simulink model "model_22"  (R2022b)
settings: Solver=ode4  StartTime=0.0  StopTime=tfinal  FixedStep=dt  RelTol=1e-3
values from neighbouring files (symbols this model uses):
  A_mat = [A_longitudinal, zeros(size(A_longitudinal,1),size(A_lateral,2)) ... (first row only)    [pre_simulink.m]
  B_mat = [B_longitudinal, zeros(size(B_longitudinal,1),2) ... (first row only)    [pre_simulink.m]
  C_mat = eye(size(A_mat))    [pre_simulink.m]
  Controls_Matrix = [0,    XDE,   XDTH,      0 ... (first row only)    [aircraft_data_reader.m]
  D_mat = zeros(size(B_mat))    [pre_simulink.m]
  dA = 0 *pi/180    (= 0)    [pre_simulink.m]
  dE = 0 *pi/180    (= 0)    [pre_simulink.m]
  dR = 0 *pi/180    (= 0)    [pre_simulink.m]
  dTH = 0    [pre_simulink.m]
  g = aircraft_data(52)    [aircraft_data_reader.m]
  Ixx = aircraft_data(53)    [aircraft_data_reader.m]
  Iyy = aircraft_data(54)    [aircraft_data_reader.m]
  Izz = aircraft_data(55)    [aircraft_data_reader.m]
  m = aircraft_data(51)    [aircraft_data_reader.m]
  mg0 = m*g * [ sin(s0(8)) ; -cos(s0(8))*sin(s0(7)) ; -cos(s0(8))*cos(s0(7)) ]    [aircraft_data_reader.m]
  s0 = aircraft_data(4:15)    [aircraft_data_reader.m]
  States_Matrix = [XU,   0,   XW,    0,   0,   0,    0 ... (first row only)    [aircraft_data_reader.m]
  U0 = s0(1)    [aircraft_data_reader.m]
undefined symbols (not defined in the file or in its folder): A_lateral_1DOF, A_lateral_2DOF, A_lateral_3DOF_DR, A_lateral_3DOF_SP, A_longitudinal_lp, A_longitudinal_sp, alpha, B_lateral_1DOF, B_lateral_2DOF, B_lateral_3DOF_DR, B_lateral_3DOF_SP, B_longitudinal_lp, B_longitudinal_sp, beta, C_lateral_1DOF, C_lateral_2DOF, C_lateral_3DOF_DR, C_lateral_3DOF_SP, C_longitudinal_lp, C_longitudinal_sp, d_a, d_e, D_lateral_1DOF, D_lateral_2DOF, D_lateral_3DOF_DR, D_lateral_3DOF_SP, D_longitudinal_lp, D_longitudinal_sp, d_r, d_th, initial_states_bus, p, phi, psi, q, r, theta, v, w, wdot, x, y, z
libraries: dspsigops x3, shared6dof x1, aerolibasang x1
settings Model: Creator=ahmed  LastModifiedBy=ahmed
settings OptimizationCC: ReuseModelBlockBuffer=on
settings DebuggingCC: SignalInfNanChecking=warning  CheckMatrixSingularityMsg=warning  SignalLabelMismatchMsg=warning  StateNameClashWarn=warning
settings RTWCC: GPUComputeCapability=5.0

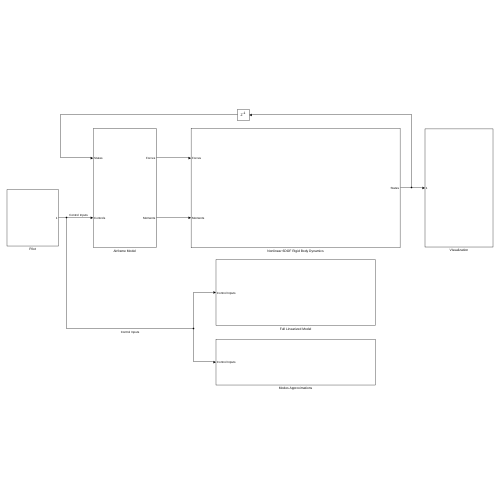
[thumbnail: Simulink's stored preview of the top-level diagram]
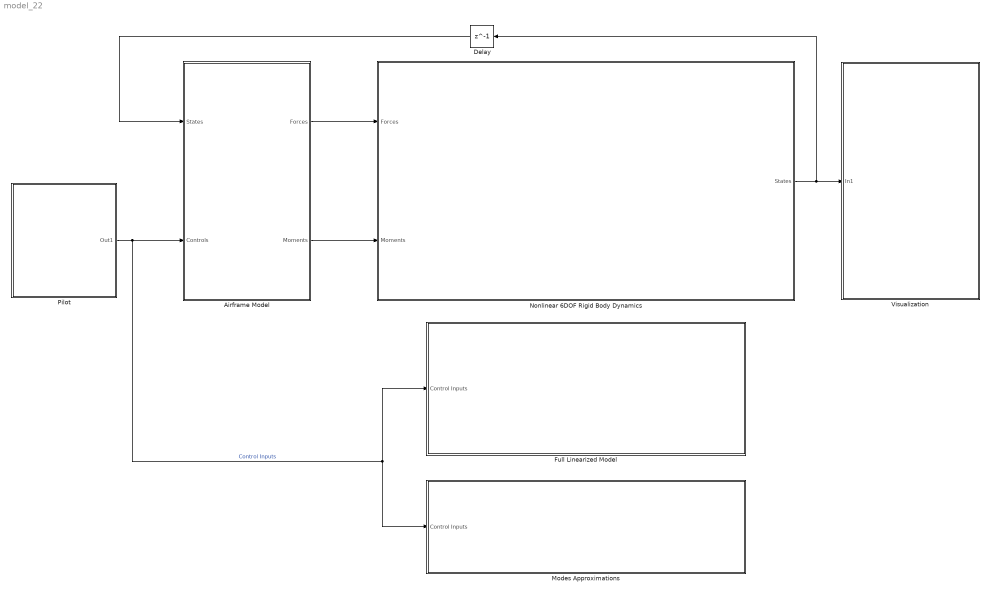
== system model_22 ==
  Airframe Model : Subsystem
  Delay : Delay  DelayLength=1  InitialCondition=initial_states_bus
  Full Linearized Model : Subsystem
  Modes Approximations : Subsystem
  Nonlinear 6DOF Rigid Body Dynamics : Subsystem
  Pilot : Subsystem
  Visualization : Subsystem
  wires:
  Airframe Model/1(Forces) -> Nonlinear 6DOF Rigid Body Dynamics/1(Forces)
  Airframe Model/2(Moments) -> Nonlinear 6DOF Rigid Body Dynamics/2(Moments)
  Nonlinear 6DOF Rigid Body Dynamics/1(States) -> Visualization/1(In1), Delay/1
  Delay/1 -> Airframe Model/1(States)
  Pilot/1(Out1) -> Modes Approximations/1(Control Inputs), Full Linearized Model/1(Control Inputs), Airframe Model/2(Controls)  "Control Inputs"

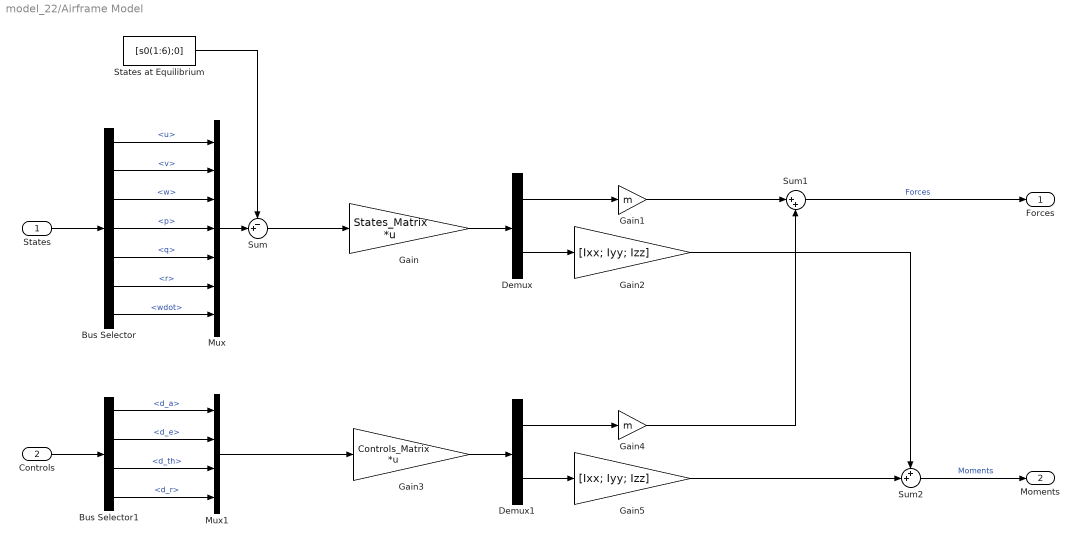
== system model_22/Airframe Model ==
  States : Inport  OutDataTypeStr=Bus: States_bus_T
  Controls : Inport  Port=2  OutDataTypeStr=Bus: Controls_bus_T
  Bus Selector : BusSelector  OutputSignals=u,v,w,p,q,r,wdot
  Bus Selector1 : BusSelector  OutputSignals=d_a,d_e,d_th,d_r
  Demux : Demux  Outputs=2
  Demux1 : Demux  Outputs=2
  Gain : Gain  Gain=States_Matrix  Multiplication=Matrix(K*u)
  Gain1 : Gain  Gain=m
  Gain2 : Gain  Gain=[Ixx; Iyy; Izz]
  Gain3 : Gain  Gain=Controls_Matrix  Multiplication=Matrix(K*u)
  Gain4 : Gain  Gain=m
  Gain5 : Gain  Gain=[Ixx; Iyy; Izz]
  Mux : Mux  Inputs=7
  Mux1 : Mux
  States at Equilibrium : Constant  Value=[s0(1:6);0]
  Sum : Sum  Inputs=-+|
  Sum1 : Sum  Inputs=|++
  Sum2 : Sum  Inputs=++|
  Forces : Outport
  Moments : Outport  Port=2
  wires:
  Sum1/1 -> Forces/1  "Forces"
  Sum2/1 -> Moments/1  "Moments"
  States/1 -> Bus Selector/1
  Bus Selector/2 -> Mux/2  "<v>"
  Bus Selector/1 -> Mux/1  "<u>"
  Bus Selector/3 -> Mux/3  "<w>"
  Bus Selector/4 -> Mux/4  "<p>"
  Bus Selector/5 -> Mux/5  "<q>"
  Bus Selector/6 -> Mux/6  "<r>"
  Bus Selector/7 -> Mux/7  "<wdot>"
  Mux/1 -> Sum/2
  States at Equilibrium/1 -> Sum/1
  Sum/1 -> Gain/1
  Gain/1 -> Demux/1
  Demux/1 -> Gain1/1
  Demux/2 -> Gain2/1
  Gain1/1 -> Sum1/1
  Gain2/1 -> Sum2/1
  Demux1/2 -> Gain5/1
  Gain3/1 -> Demux1/1
  Controls/1 -> Bus Selector1/1
  Bus Selector1/3 -> Mux1/3  "<d_th>"
  Bus Selector1/2 -> Mux1/2  "<d_e>"
  Bus Selector1/1 -> Mux1/1  "<d_a>"
  Bus Selector1/4 -> Mux1/4  "<d_r>"
  Mux1/1 -> Gain3/1
  Gain5/1 -> Sum2/2
  Demux1/1 -> Gain4/1
  Gain4/1 -> Sum1/2

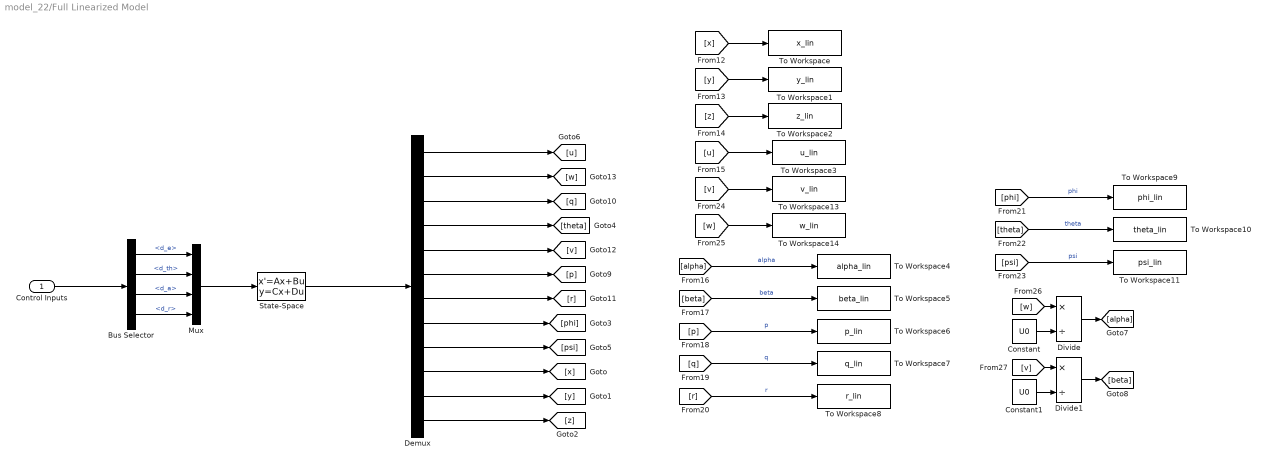
== system model_22/Full Linearized Model ==
  Control Inputs : Inport
  Bus Selector : BusSelector  OutputSignals=d_e,d_th,d_a,d_r
  Constant : Constant  Value=U0
  Constant1 : Constant  Value=U0
  Demux : Demux  Outputs=12
  Divide : Product  Inputs=*/
  Divide1 : Product  Inputs=*/
  Mux : Mux
  State-Space : StateSpace  A=A_mat  B=B_mat  C=C_mat  D=D_mat  InitialCondition=[s0(1); s0(3); s0(5); s0(8); s0(2); s0(4); s0(6); s0(7); s0(9:12)]
  To Workspace : ToWorkspace  VariableName=x_lin  SaveFormat=Timeseries  SampleTime=-1
  To Workspace1 : ToWorkspace  VariableName=y_lin  SaveFormat=Timeseries  SampleTime=-1
  To Workspace10 : ToWorkspace  VariableName=theta_lin  SaveFormat=Timeseries  SampleTime=-1
  To Workspace11 : ToWorkspace  VariableName=psi_lin  SaveFormat=Timeseries  SampleTime=-1
  To Workspace13 : ToWorkspace  VariableName=v_lin  SaveFormat=Timeseries  SampleTime=-1
  To Workspace14 : ToWorkspace  VariableName=w_lin  SaveFormat=Timeseries  SampleTime=-1
  To Workspace2 : ToWorkspace  VariableName=z_lin  SaveFormat=Timeseries  SampleTime=-1
  To Workspace3 : ToWorkspace  VariableName=u_lin  SaveFormat=Timeseries  SampleTime=-1
  To Workspace4 : ToWorkspace  VariableName=alpha_lin  SaveFormat=Timeseries  SampleTime=-1
  To Workspace5 : ToWorkspace  VariableName=beta_lin  SaveFormat=Timeseries  SampleTime=-1
  To Workspace6 : ToWorkspace  VariableName=p_lin  SaveFormat=Timeseries  SampleTime=-1
  To Workspace7 : ToWorkspace  VariableName=q_lin  SaveFormat=Timeseries  SampleTime=-1
  To Workspace8 : ToWorkspace  VariableName=r_lin  SaveFormat=Timeseries  SampleTime=-1
  To Workspace9 : ToWorkspace  VariableName=phi_lin  SaveFormat=Timeseries  SampleTime=-1
  wires:
  Bus Selector/4 -> Mux/4  "<d_r>"
  Bus Selector/1 -> Mux/1  "<d_e>"
  Bus Selector/2 -> Mux/2  "<d_th>"
  Mux/1 -> State-Space/1
  Bus Selector/3 -> Mux/3  "<d_a>"
  State-Space/1 -> Demux/1
  Control Inputs/1 -> Bus Selector/1
  [theta] -> To Workspace10/1  "theta"
  Demux/6 -> [p]
  Demux/5 -> [v]
  Demux/4 -> [theta]
  [alpha] -> To Workspace4/1  "alpha"
  Demux/2 -> [w]
  Constant/1 -> Divide/2
  Demux/3 -> [q]
  Demux/7 -> [r]
  Divide/1 -> [alpha]
  [w] -> Divide/1
  [p] -> To Workspace6/1  "p"
  [beta] -> To Workspace5/1  "beta"
  Demux/9 -> [psi]
  [psi] -> To Workspace11/1  "psi"
  [v] -> To Workspace13/1
  Divide1/1 -> [beta]
  [v] -> Divide1/1
  [q] -> To Workspace7/1  "q"
  Demux/10 -> [x]
  [u] -> To Workspace3/1
  [r] -> To Workspace8/1  "r"
  [w] -> To Workspace14/1
  [z] -> To Workspace2/1
  [phi] -> To Workspace9/1  "phi"
  Demux/12 -> [z]
  Demux/1 -> [u]
  Demux/8 -> [phi]
  Constant1/1 -> Divide1/2
  [x] -> To Workspace/1
  Demux/11 -> [y]
  [y] -> To Workspace1/1

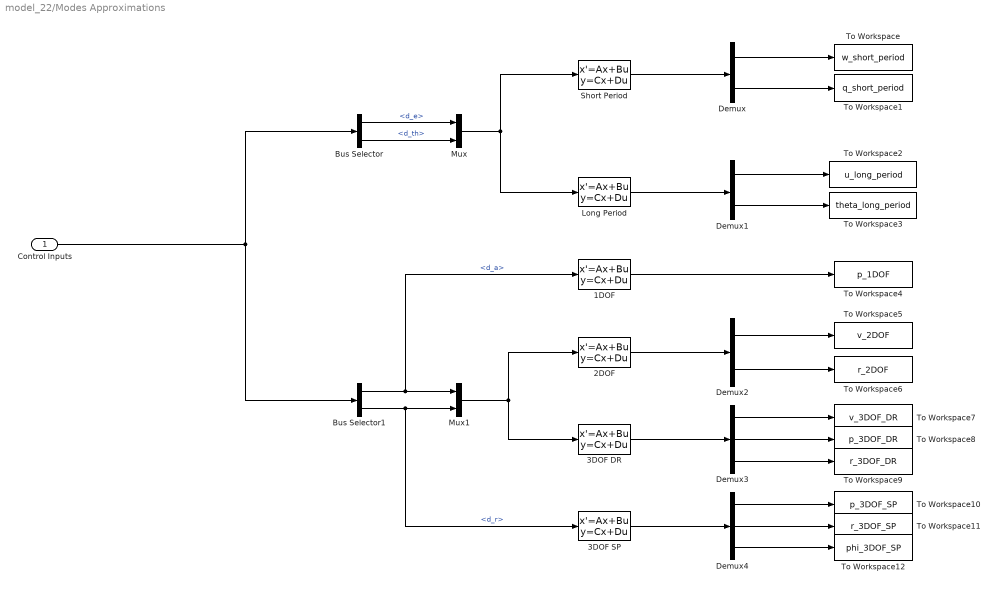
== system model_22/Modes Approximations ==
  Control Inputs : Inport
  1DOF : StateSpace  A=A_lateral_1DOF  B=B_lateral_1DOF  C=C_lateral_1DOF  D=D_lateral_1DOF  InitialCondition=s0(4)
  2DOF : StateSpace  A=A_lateral_2DOF  B=B_lateral_2DOF  C=C_lateral_2DOF  D=D_lateral_2DOF  InitialCondition=[s0(2); s0(6)]
  3DOF DR : StateSpace  A=A_lateral_3DOF_DR  B=B_lateral_3DOF_DR  C=C_lateral_3DOF_DR  D=D_lateral_3DOF_DR  InitialCondition=[s0(2); s0(4); s0(6)]
  3DOF SP : StateSpace  A=A_lateral_3DOF_SP  B=B_lateral_3DOF_SP  C=C_lateral_3DOF_SP  D=D_lateral_3DOF_SP  InitialCondition=[s0(4); s0(6); s0(7)]
  Bus Selector : BusSelector  OutputSignals=d_e,d_th
  Bus Selector1 : BusSelector  OutputSignals=d_a,d_r
  Demux : Demux  Outputs=2
  Demux1 : Demux  Outputs=2
  Demux2 : Demux  Outputs=2
  Demux3 : Demux  Outputs=3
  Demux4 : Demux  Outputs=3
  Long Period : StateSpace  A=A_longitudinal_lp  B=B_longitudinal_lp  C=C_longitudinal_lp  D=D_longitudinal_lp  InitialCondition=[s0(1); s0(8)]
  Mux : Mux  Inputs=2
  Mux1 : Mux  Inputs=2
  Short Period : StateSpace  A=A_longitudinal_sp  B=B_longitudinal_sp  C=C_longitudinal_sp  D=D_longitudinal_sp  InitialCondition=[s0(3); s0(5)]
  To Workspace : ToWorkspace  VariableName=w_short_period  SaveFormat=Timeseries  SampleTime=-1
  To Workspace1 : ToWorkspace  VariableName=q_short_period  SaveFormat=Timeseries  SampleTime=-1
  To Workspace10 : ToWorkspace  VariableName=p_3DOF_SP  SaveFormat=Timeseries  SampleTime=-1
  To Workspace11 : ToWorkspace  VariableName=r_3DOF_SP  SaveFormat=Timeseries  SampleTime=-1
  To Workspace12 : ToWorkspace  VariableName=phi_3DOF_SP  SaveFormat=Timeseries  SampleTime=-1
  To Workspace2 : ToWorkspace  VariableName=u_long_period  SaveFormat=Timeseries  SampleTime=-1
  To Workspace3 : ToWorkspace  VariableName=theta_long_period  SaveFormat=Timeseries  SampleTime=-1
  To Workspace4 : ToWorkspace  VariableName=p_1DOF  SaveFormat=Timeseries  SampleTime=-1
  To Workspace5 : ToWorkspace  VariableName=v_2DOF  SaveFormat=Timeseries  SampleTime=-1
  To Workspace6 : ToWorkspace  VariableName=r_2DOF  SaveFormat=Timeseries  SampleTime=-1
  To Workspace7 : ToWorkspace  VariableName=v_3DOF_DR  SaveFormat=Timeseries  SampleTime=-1
  To Workspace8 : ToWorkspace  VariableName=p_3DOF_DR  SaveFormat=Timeseries  SampleTime=-1
  To Workspace9 : ToWorkspace  VariableName=r_3DOF_DR  SaveFormat=Timeseries  SampleTime=-1
  wires:
  Demux4/2 -> To Workspace11/1
  Bus Selector1/1 -> 1DOF/1, Mux1/1  "<d_a>"
  Demux1/1 -> To Workspace2/1
  Demux3/2 -> To Workspace8/1
  Demux3/3 -> To Workspace9/1
  Demux2/1 -> To Workspace5/1
  Demux2/2 -> To Workspace6/1
  3DOF SP/1 -> Demux4/1
  Mux1/1 -> 3DOF DR/1, 2DOF/1
  Short Period/1 -> Demux/1
  Demux3/1 -> To Workspace7/1
  Demux4/1 -> To Workspace10/1
  Demux1/2 -> To Workspace3/1
  Control Inputs/1 -> Bus Selector/1, Bus Selector1/1
  Long Period/1 -> Demux1/1
  Demux4/3 -> To Workspace12/1
  1DOF/1 -> To Workspace4/1
  Bus Selector1/2 -> 3DOF SP/1, Mux1/2  "<d_r>"
  3DOF DR/1 -> Demux3/1
  Demux/1 -> To Workspace/1
  2DOF/1 -> Demux2/1
  Bus Selector/2 -> Mux/2  "<d_th>"
  Mux/1 -> Long Period/1, Short Period/1
  Demux/2 -> To Workspace1/1
  Bus Selector/1 -> Mux/1  "<d_e>"

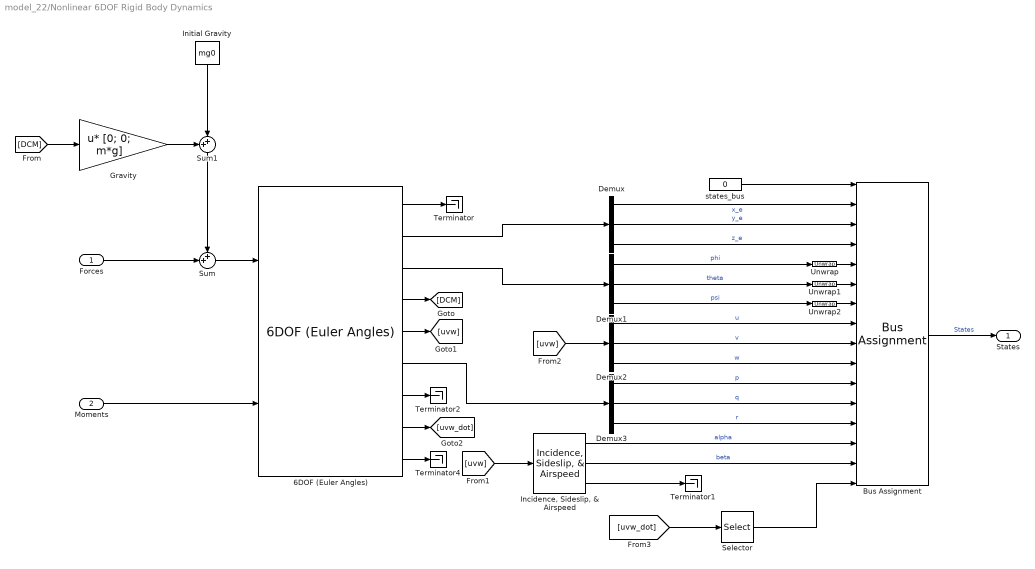
== system model_22/Nonlinear 6DOF Rigid Body Dynamics ==
  Forces : Inport
  Moments : Inport  Port=2
  6DOF (Euler Angles) : shared6dof/6DOF (Euler Angles)  units=English (Velocity in ft/s)  mtype=Fixed  rep=Euler Angles  xme_0=s0(10:12)  Vm_0=s0(1:3)  eul_0=s0(7:9)  pm_0=s0(4:6)  mass_0=m  mass_e=0.5  mass_f=2.0  inertia=I  inertia_e=eye(3)  inertia_f=2*eye(3)  k_quat=1.0  vre_flag=on  abi_flag=on  aMode=0  xme_statename=''  Vm_statename=''  eul_statename=''  quat_statename=''  pm_statename=''  mass_statename=''
  Bus Assignment : BusAssignment  AssignedSignals=x,y,z,phi,theta,psi,u,v,w,p,q,r,alpha,beta,wdot
  Demux{,1..3} (4 alike) : Demux  Outputs=3
  Gravity : Gain  Gain=[0; 0; m*g]  Multiplication=Matrix(u*K)
  "Incidence, Sideslip, & Airspeed" : aerolibasang/Incidence, Sideslip, & Airspeed
  Initial Gravity : Constant  Value=mg0
  Selector : Selector  InputPortWidth=3  IndexOptions=Index vector (dialog)  Indices=3  OutputSizes=1
  Sum : Sum  Inputs=++|
  Sum1 : Sum  Inputs=++|
  Terminator{,1..2,4} (4 alike) : Terminator
  Unwrap : dspsigops/Unwrap  tol=pi  running=off
  Unwrap1 : dspsigops/Unwrap  tol=pi  running=off
  Unwrap2 : dspsigops/Unwrap  tol=pi  running=off
  states_bus : Constant  Value=0  OutDataTypeStr=Bus: States_bus_T  SampleTime=-1
  States : Outport  OutDataTypeStr=Bus: States_bus_T
  wires:
  Bus Assignment/1 -> States/1  "States"
  Demux1/2 -> Unwrap1/1  "theta"
  Demux3/2 -> Bus Assignment/12  "q"
  6DOF (Euler Angles)/7 -> Terminator2/1
  6DOF (Euler Angles)/1 -> Terminator/1
  6DOF (Euler Angles)/3 -> Demux1/1
  states_bus/1 -> Bus Assignment/1
  Forces/1 -> Sum/2
  6DOF (Euler Angles)/6 -> Demux3/1
  6DOF (Euler Angles)/8 -> [uvw_dot]
  Demux2/2 -> Bus Assignment/9  "v"
  Demux1/3 -> Unwrap2/1  "psi"
  Demux3/3 -> Bus Assignment/13  "r"
  Demux2/1 -> Bus Assignment/8  "u"
  Demux2/3 -> Bus Assignment/10  "w"
  6DOF (Euler Angles)/2 -> Demux/1
  Demux/3 -> Bus Assignment/4  "z_e"
  Demux1/1 -> Unwrap/1  "phi"
  Demux/2 -> Bus Assignment/3  "y_e"
  Demux/1 -> Bus Assignment/2  "x_e"
  6DOF (Euler Angles)/9 -> Terminator4/1
  Demux3/1 -> Bus Assignment/11  "p"
  6DOF (Euler Angles)/4 -> [DCM]
  Unwrap/1 -> Bus Assignment/5
  Unwrap1/1 -> Bus Assignment/6
  Unwrap2/1 -> Bus Assignment/7
  [DCM] -> Gravity/1
  Gravity/1 -> Sum1/1
  Initial Gravity/1 -> Sum1/2
  Sum1/1 -> Sum/1
  Sum/1 -> 6DOF (Euler Angles)/1
  6DOF (Euler Angles)/5 -> [uvw]
  [uvw] -> "Incidence, Sideslip, & Airspeed"/1
  "Incidence, Sideslip, & Airspeed"/3 -> Terminator1/1
  "Incidence, Sideslip, & Airspeed"/2 -> Bus Assignment/15  "beta"
  "Incidence, Sideslip, & Airspeed"/1 -> Bus Assignment/14  "alpha"
  [uvw] -> Demux2/1
  Moments/1 -> 6DOF (Euler Angles)/2
  [uvw_dot] -> Selector/1
  Selector/1 -> Bus Assignment/16

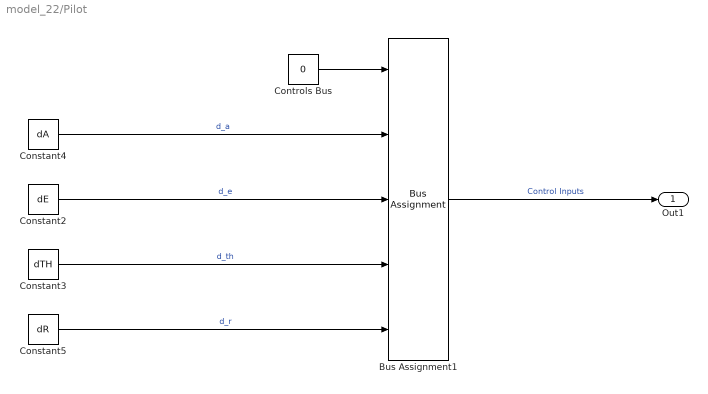
== system model_22/Pilot ==
  Bus Assignment1 : BusAssignment  AssignedSignals=d_a,d_e,d_th,d_r
  Constant2 : Constant  Value=dE
  Constant3 : Constant  Value=dTH
  Constant4 : Constant  Value=dA
  Constant5 : Constant  Value=dR
  Controls Bus : Constant  Value=0  OutDataTypeStr=Bus: Controls_bus_T
  Out1 : Outport
  wires:
  Constant2/1 -> Bus Assignment1/3  "d_e"
  Constant4/1 -> Bus Assignment1/2  "d_a"
  Constant5/1 -> Bus Assignment1/5  "d_r"
  Constant3/1 -> Bus Assignment1/4  "d_th"
  Controls Bus/1 -> Bus Assignment1/1
  Bus Assignment1/1 -> Out1/1  "Control Inputs"

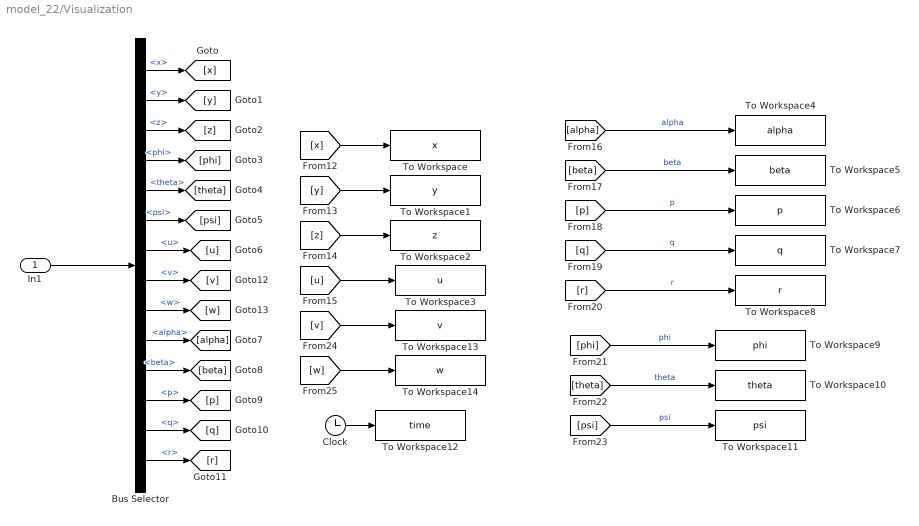
== system model_22/Visualization ==
  In1 : Inport
  Bus Selector : BusSelector  OutputSignals=x,y,z,phi,theta,psi,u,v,w,alpha,beta,p,q,r
  Clock : Clock
  To Workspace : ToWorkspace  VariableName=x  SaveFormat=Timeseries  SampleTime=-1
  To Workspace1 : ToWorkspace  VariableName=y  SaveFormat=Timeseries  SampleTime=-1
  To Workspace10 : ToWorkspace  VariableName=theta  SaveFormat=Timeseries  SampleTime=-1
  To Workspace11 : ToWorkspace  VariableName=psi  SaveFormat=Timeseries  SampleTime=-1
  To Workspace12 : ToWorkspace  VariableName=time  SaveFormat=Timeseries  SampleTime=-1
  To Workspace13 : ToWorkspace  VariableName=v  SaveFormat=Timeseries  SampleTime=-1
  To Workspace14 : ToWorkspace  VariableName=w  SaveFormat=Timeseries  SampleTime=-1
  To Workspace2 : ToWorkspace  VariableName=z  SaveFormat=Timeseries  SampleTime=-1
  To Workspace3 : ToWorkspace  VariableName=u  SaveFormat=Timeseries  SampleTime=-1
  To Workspace4 : ToWorkspace  VariableName=alpha  SaveFormat=Timeseries  SampleTime=-1
  To Workspace5 : ToWorkspace  VariableName=beta  SaveFormat=Timeseries  SampleTime=-1
  To Workspace6 : ToWorkspace  VariableName=p  SaveFormat=Timeseries  SampleTime=-1
  To Workspace7 : ToWorkspace  VariableName=q  SaveFormat=Timeseries  SampleTime=-1
  To Workspace8 : ToWorkspace  VariableName=r  SaveFormat=Timeseries  SampleTime=-1
  To Workspace9 : ToWorkspace  VariableName=phi  SaveFormat=Timeseries  SampleTime=-1
  wires:
  Bus Selector/6 -> [psi]  "<psi>"
  Bus Selector/1 -> [x]  "<x>"
  Bus Selector/7 -> [u]  "<u>"
  Bus Selector/4 -> [phi]  "<phi>"
  Bus Selector/10 -> [alpha]  "<alpha>"
  Bus Selector/14 -> [r]  "<r>"
  Bus Selector/11 -> [beta]  "<beta>"
  Bus Selector/5 -> [theta]  "<theta>"
  Bus Selector/13 -> [q]  "<q>"
  Bus Selector/12 -> [p]  "<p>"
  Bus Selector/2 -> [y]  "<y>"
  Bus Selector/3 -> [z]  "<z>"
  In1/1 -> Bus Selector/1
  [x] -> To Workspace/1
  [y] -> To Workspace1/1
  [z] -> To Workspace2/1
  [u] -> To Workspace3/1
  Clock/1 -> To Workspace12/1
  [phi] -> To Workspace9/1  "phi"
  [theta] -> To Workspace10/1  "theta"
  [psi] -> To Workspace11/1  "psi"
  [alpha] -> To Workspace4/1  "alpha"
  [beta] -> To Workspace5/1  "beta"
  [p] -> To Workspace6/1  "p"
  [q] -> To Workspace7/1  "q"
  [r] -> To Workspace8/1  "r"
  [v] -> To Workspace13/1
  Bus Selector/8 -> [v]  "<v>"
  Bus Selector/9 -> [w]  "<w>"
  [w] -> To Workspace14/1
